simulink model "Aero2_Workspace"  (R2023a)
settings: Solver=ode4  StartTime=0.0  StopTime=inf  FixedStep=0.001  RelTol=1e-3  EnableMultiTasking=on
model workspace (MAT data in the model file):
  Dp = 0.001964
  Dt = 0.16743
  Dy = 0.001776
  Fc_p = 0
  Fc_y = 0.000919
  Jm = 4e-06
  Jp = 0.02318850045
  Jr = 4.4030375e-05
  Jr_p = 1.626e-05
  Jy = 0.02381041595
  Ka_p = 2.054e-06
  Ka_y = 1.1752e-06
  Ksp = 0.012956
  Rm = 10.6
  Sig = Simulink.Signal
  Sig.DataType = 'auto'
  Sig.Dimensions = -1
  Sig.DimensionsMode = 'auto'
  Sig.Complexity = 'auto'
  Sig.SampleTime = -1
  Sig.SamplingMode = 'auto'
  km = 0.04
  kt = 0.04
undefined symbols (not defined in the file or in its folder): qc_get_step_size
libraries: quarc_library x10, simulink x4
settings Model: SimulationMode=external  ExtModeTrigDuration=10000  Creator=mbohra  LastModifiedBy=Derek
settings SolverCC: AlgebraicLoopSolver=TrustRegion  PositivePriorityOrder=on
settings DataIOCC: ReturnWorkspaceOutputs=off
settings OptimizationCC: ReuseModelBlockBuffer=off
settings DebuggingCC: UnconnectedInputMsg=warning  UnconnectedOutputMsg=warning  UnconnectedLineMsg=warning  ArithmeticOperatorsInVariantConditions=warning
settings ModelReferenceCC: EnableRefExpFcnMdlSchedulingChecks=on
settings SFSimCC: SimUseLocalCustomCode=off  CustomCodeUndefinedFunction=UseInterfaceOnly
settings RTWCC: Description=QUARC Win64 Target Using Toolchain  SystemTargetFile=quarc_win64.tlc  TemplateMakefile=quarc_default_tmf  PostCodeGenCommand=packNGo(buildInfo, 'packType', 'hierarchical')  RTWUseLocalCustomCode=off  Toolchain=QUARC win64 | nmake (64-bit Windows)  BuildConfiguration=Faster Runs  DLArmComputeVersion=19.05
settings CodeAppCC: StateflowObjectComments=on
settings STFCustomTargetCC: SystemTargetFile=quarc_win64.tlc
settings GRTTargetCC: ParMdlRefBuildCompliant=off  CompOptLevelCompliant=off  CombineOutputUpdateFcns=off  MatFileLogging=off  CPPClassGenCompliant=off  GRTInterface=on  ExtMode=on  ExtModeMexFile=quarc_comm
settings ConfigComp: CovMetricSettings=dswe

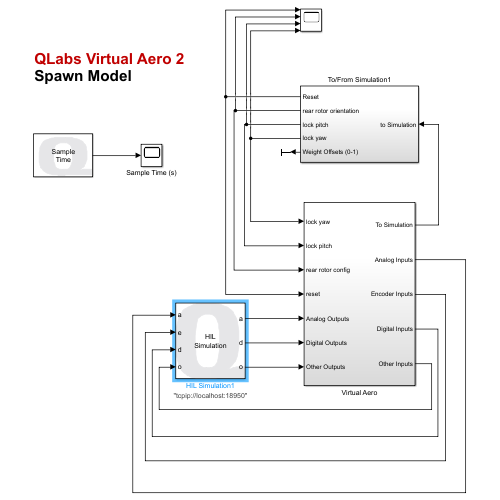
[thumbnail: Simulink's stored preview of the top-level diagram]
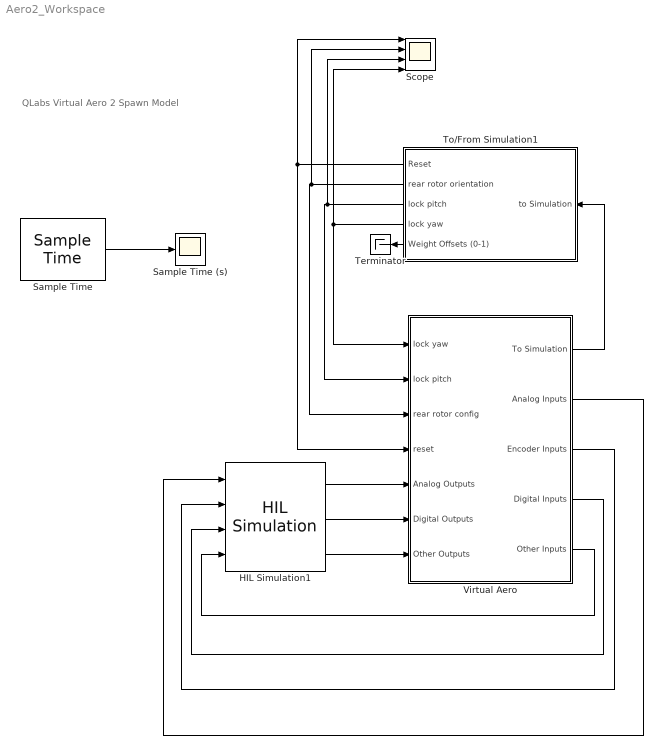
== system Aero2_Workspace ==
  note: QLabs Virtual Aero 2
      | Spawn Model
  HIL Simulation1 : quarc_library/Data Acquisition/Generic/Configuration/HIL Simulation  uri_source=Specify via dialog (do not evaluate)  uri=tcpip://localhost:18950  board_type=quanser_aero2_usb  board_id=0  sample_time=qc_get_step_size  active=on  num_clocks=1  num_interrupts=0  num_analog_inputs=2  num_analog_outputs=2  initial_analog=[]  num_digital_io=0  num_digital_inputs=3  num_digital_outputs=2  initial_digital=[1 1]  num_encoder_inputs=4  num_pwm_outputs=0  initial_pwm=[]  other_inputs=[3000:3002 4000:4002 14000:14003]  other_outputs=[11000:11002]  initial_other=[]  integer_get_property_codes=[]  double_get_property_codes=[]  string_get_property_codes=[]  integer_set_property_codes=[]  double_set_property_codes=[]  string_set_property_codes=[]  initial_integer_properties=0  initial_double_properties=0  initial_string_properties=[]  max_string_property=80  use_variable_size_strings=off
      settings: AttributesFormatString="\"tcpip://localhost:18950\""  SourceProductName=QUARC Targets
  Sample Time : quarc_library/Sources/Time/Sample Time  Priority=-99  sample_time=qc_get_step_size
  Sample Time (s) : Scope
  Scope : Scope  NumInputPorts=4
  Terminator : Terminator
  To/From Simulation1 : Subsystem
  Virtual Aero : Subsystem
  wires:
  HIL Simulation1/1 -> Virtual Aero/5(Analog Outputs)
  HIL Simulation1/2 -> Virtual Aero/6(Digital Outputs)
  HIL Simulation1/3 -> Virtual Aero/7(Other Outputs)
  Virtual Aero/5(Other Inputs) -> HIL Simulation1/4
  Virtual Aero/3(Encoder Inputs) -> HIL Simulation1/2
  Virtual Aero/2(Analog Inputs) -> HIL Simulation1/1
  To/From Simulation1/4(lock yaw) -> Virtual Aero/1(lock yaw), Scope/4
  To/From Simulation1/3(lock pitch) -> Scope/3, Virtual Aero/2(lock pitch)
  To/From Simulation1/1(Reset) -> Scope/1, Virtual Aero/4(reset)
  To/From Simulation1/2(rear rotor orientation) -> Scope/2, Virtual Aero/3(rear rotor config)
  Sample Time/1 -> Sample Time (s)/1
  Virtual Aero/1(To Simulation) -> To/From Simulation1/1(to Simulation)
  To/From Simulation1/5(Weight Offsets (0-1)) -> Terminator/1
  Virtual Aero/4(Digital Inputs) -> HIL Simulation1/3

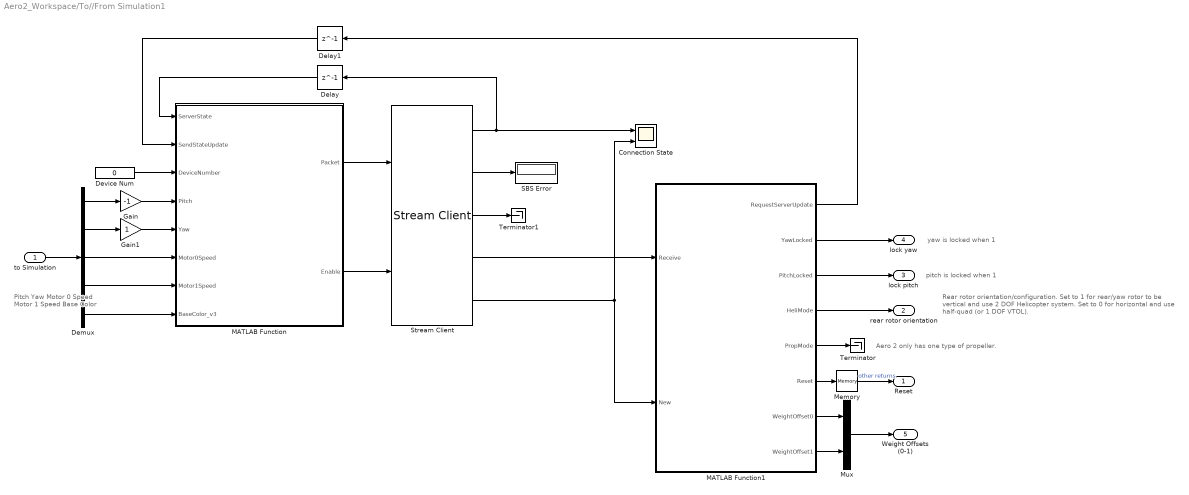
== system Aero2_Workspace/To//From Simulation1 ==
  note: Aero 2 only has one type of propeller.
  note: pitch is locked when 1
  note: Pitch
      | Yaw
      | Motor 0 Speed
      | Motor 1 Speed
      | Base Color
  note: Rear rotor orientation/configuration.
      | Set to 1 for rear/yaw rotor to be vertical and use 2 DOF Helicopter system.
      | Set to 0 for horizontal and use half-quad (or 1 DOF VTOL).
  note: yaw is locked when 1
  to Simulation : Inport
  "Connection State " : Scope  NumInputPorts=2
  Delay : Delay  DelayLength=1
  Delay1 : Delay  DelayLength=1
  Demux : Demux  Outputs=[1 1 1 1 3]
  Device Num : Constant  Value=0
  Gain : Gain  Gain=-1
  Gain1 : Gain
  MATLAB Function : MATLAB Function  TreatAsAtomicUnit=on
  MATLAB Function1 : MATLAB Function  TreatAsAtomicUnit=on
  Memory : Memory
  Mux : Mux  Inputs=2
  SBS Error : Display
      settings: Decimation=20
  Stream Client : quarc_library/Communications/Basic/Stream Client  uri_source=Specify via dialog (do not evaluate)  uri=tcpip://localhost:18000?nagle='off'  send_buffer_size=65537  receive_buffer_size=65537  byte_order=little endian (Intel - LSB first)  optimization=Minimum latency  send_options=Send all data  receive_options=Receive all data  default_value=[0]  sample_time=qc_get_step_size  active=off  implementation=Use blocking I/O in a separate thread  send_fifo_size=3  receive_fifo_size=3  send_priority=0  receive_priority=0  send_dimensions=on  receive_dimensions=on  max_dimensions=65537  data_type=uint8  type_expr=BusObject
      settings: AttributesFormatString="\"tcpip://localhost:18000?nagle='off'\""
  Terminator : Terminator
  Terminator1 : Terminator
  Reset : Outport  VectorParamsAs1DForOutWhenUnconnected=off
  rear rotor orientation : Outport  Port=2  VectorParamsAs1DForOutWhenUnconnected=off
  lock pitch : Outport  Port=3  VectorParamsAs1DForOutWhenUnconnected=off
  lock yaw : Outport  Port=4  VectorParamsAs1DForOutWhenUnconnected=off
  Weight Offsets (0-1) : Outport  Port=5  OutDataTypeStr=double  VectorParamsAs1DForOutWhenUnconnected=off
  wires:
  MATLAB Function1/3(PitchLocked) -> lock pitch/1
  MATLAB Function1/2(YawLocked) -> lock yaw/1
  MATLAB Function1/4(HeliMode) -> rear rotor orientation/1
  MATLAB Function/1(Packet) -> Stream Client/1
  Stream Client/5 -> MATLAB Function1/2(New), "Connection State "/2
  Stream Client/2 -> SBS Error/1
  Demux/5 -> MATLAB Function/8(BaseColor_v3)
  Stream Client/4 -> MATLAB Function1/1(Receive)
  Stream Client/3 -> Terminator1/1
  Demux/4 -> MATLAB Function/7(Motor1Speed)
  MATLAB Function/2(Enable) -> Stream Client/2
  Demux/3 -> MATLAB Function/6(Motor0Speed)
  MATLAB Function1/1(RequestServerUpdate) -> Delay1/1
  to Simulation/1 -> Demux/1
  Delay1/1 -> MATLAB Function/2(SendStateUpdate)
  Stream Client/1 -> Delay/1, "Connection State "/1
  Delay/1 -> MATLAB Function/1(ServerState)
  Device Num/1 -> MATLAB Function/3(DeviceNumber)
  Demux/1 -> Gain/1
  Demux/2 -> Gain1/1
  MATLAB Function1/6(Reset) -> Memory/1
  MATLAB Function1/5(PropMode) -> Terminator/1
  Mux/1 -> Weight Offsets (0-1)/1
  MATLAB Function1/7(WeightOffset0) -> Mux/1
  MATLAB Function1/8(WeightOffset1) -> Mux/2
  Memory/1 -> Reset/1  "other returns"
  Gain/1 -> MATLAB Function/4(Pitch)
  Gain1/1 -> MATLAB Function/5(Yaw)

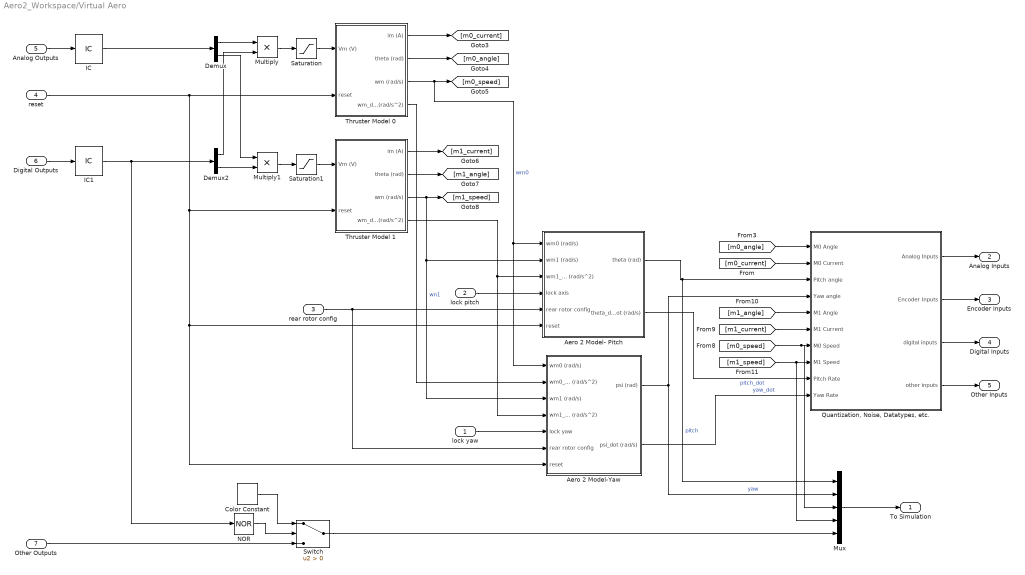
== system Aero2_Workspace/Virtual Aero ==
  lock yaw : Inport
  lock pitch : Inport  Port=2
  rear rotor config : Inport  Port=3
  reset : Inport  Port=4
  Analog Outputs : Inport  Port=5
  Digital Outputs : Inport  Port=6
  Other Outputs : Inport  Port=7
  Aero 2 Model- Pitch : Subsystem
  Aero 2 Model-Yaw : Subsystem
  Color Constant : quarc_library/Sources/Signals/Color Constant  color=[1 0 0]
      settings: SourceProductName=QUARC Targets
  Demux : Demux  Outputs=2
  Demux2 : Demux  Outputs=2
  IC : InitialCondition  Value=0
  IC1 : InitialCondition  Value=0
  Multiply : Product
  Multiply1 : Product
  Mux : Mux  Inputs=5
  NOR : Logic  Operator=NOR  Inputs=1  IconShape=distinctive  AllPortsSameDT=off  OutDataTypeStr=boolean
  "Quantization, Noise, Datatypes, etc." : Subsystem
  Saturation : Saturate  UpperLimit=24  LowerLimit=-24
  Saturation1 : Saturate  UpperLimit=24  LowerLimit=-24
  Switch : Switch  Criteria=u2 > Threshold  SaturateOnIntegerOverflow=off  InputSameDT=off
  Thruster Model 0 : Subsystem
  Thruster Model 1 : Subsystem
  To Simulation : Outport  VectorParamsAs1DForOutWhenUnconnected=off
  Analog Inputs : Outport  Port=2  VectorParamsAs1DForOutWhenUnconnected=off
  Encoder Inputs : Outport  Port=3  VectorParamsAs1DForOutWhenUnconnected=off
  Digital Inputs : Outport  Port=4  VectorParamsAs1DForOutWhenUnconnected=off
  Other Inputs : Outport  Port=5  VectorParamsAs1DForOutWhenUnconnected=off
  wires:
  Analog Outputs/1 -> IC/1
  Digital Outputs/1 -> IC1/1
  Demux/1 -> Multiply/1
  Demux2/1 -> Multiply/2
  Demux/2 -> Multiply1/1
  Demux2/2 -> Multiply1/2
  "Quantization, Noise, Datatypes, etc."/1(Analog Inputs) -> Analog Inputs/1
  "Quantization, Noise, Datatypes, etc."/2(Encoder Inputs) -> Encoder Inputs/1
  "Quantization, Noise, Datatypes, etc."/4(other inputs) -> Other Inputs/1
  Thruster Model 0/1(im (A)) -> [m0_current]
  Thruster Model 0/2(theta (rad)) -> [m0_angle]
  Thruster Model 0/3(wm (rad/s)) -> [m0_speed], Aero 2 Model-Yaw/1(wm0 (rad/s)), Aero 2 Model- Pitch/1(wm0 (rad/s))  "wm0"
  [m0_current] -> "Quantization, Noise, Datatypes, etc."/2(M0 Current)
  [m0_angle] -> "Quantization, Noise, Datatypes, etc."/1(M0 Angle)
  [m0_speed] -> Mux/3, "Quantization, Noise, Datatypes, etc."/7(M0 Speed)
  [m1_speed] -> "Quantization, Noise, Datatypes, etc."/8(M1 Speed), Mux/4
  [m1_angle] -> "Quantization, Noise, Datatypes, etc."/5(M1 Angle)
  [m1_current] -> "Quantization, Noise, Datatypes, etc."/6(M1 Current)
  Aero 2 Model-Yaw/1(psi (rad)) -> "Quantization, Noise, Datatypes, etc."/4(Yaw angle), Mux/2  "yaw"
  Thruster Model 1/1(im (A)) -> [m1_current]
  Thruster Model 1/2(theta (rad)) -> [m1_angle]
  Thruster Model 1/3(wm (rad/s)) -> Aero 2 Model-Yaw/3(wm1 (rad/s)), Aero 2 Model- Pitch/2(wm1 (rad/s)), [m1_speed]  "wn1"
  Thruster Model 0/4(wm_dot (rad/s^2)) -> Aero 2 Model-Yaw/2(wm0_dot (rad/s^2))
  Aero 2 Model-Yaw/2(psi_dot (rad/s)) -> "Quantization, Noise, Datatypes, etc."/10(Yaw Rate)  "yaw_dot"
  Thruster Model 1/4(wm_dot (rad/s^2)) -> Aero 2 Model-Yaw/4(wm1_dot (rad/s^2)), Aero 2 Model- Pitch/3(wm1_dot (rad/s^2))
  lock yaw/1 -> Aero 2 Model-Yaw/5(lock yaw)
  lock pitch/1 -> Aero 2 Model- Pitch/4(lock axis)
  reset/1 -> Thruster Model 1/2(reset), Aero 2 Model- Pitch/6(reset), Aero 2 Model-Yaw/7(reset), Thruster Model 0/2(reset)
  rear rotor config/1 -> Aero 2 Model-Yaw/6(rear rotor config), Aero 2 Model- Pitch/5(rear rotor config)
  IC1/1 -> Demux2/1, NOR/1
  Multiply/1 -> Saturation/1
  Saturation/1 -> Thruster Model 0/1(Vm (V))
  Multiply1/1 -> Saturation1/1
  Saturation1/1 -> Thruster Model 1/1(Vm (V))
  Aero 2 Model- Pitch/1(theta (rad)) -> Mux/1, "Quantization, Noise, Datatypes, etc."/3(Pitch angle)  "pitch"
  Aero 2 Model- Pitch/2(theta_dot (rad/s)) -> "Quantization, Noise, Datatypes, etc."/9(Pitch Rate)  "pitch_dot"
  Mux/1 -> To Simulation/1
  "Quantization, Noise, Datatypes, etc."/3(digital inputs) -> Digital Inputs/1
  Color Constant/1 -> Switch/1
  NOR/1 -> Switch/2
  Other Outputs/1 -> Switch/3
  Switch/1 -> Mux/5
  IC/1 -> Demux/1

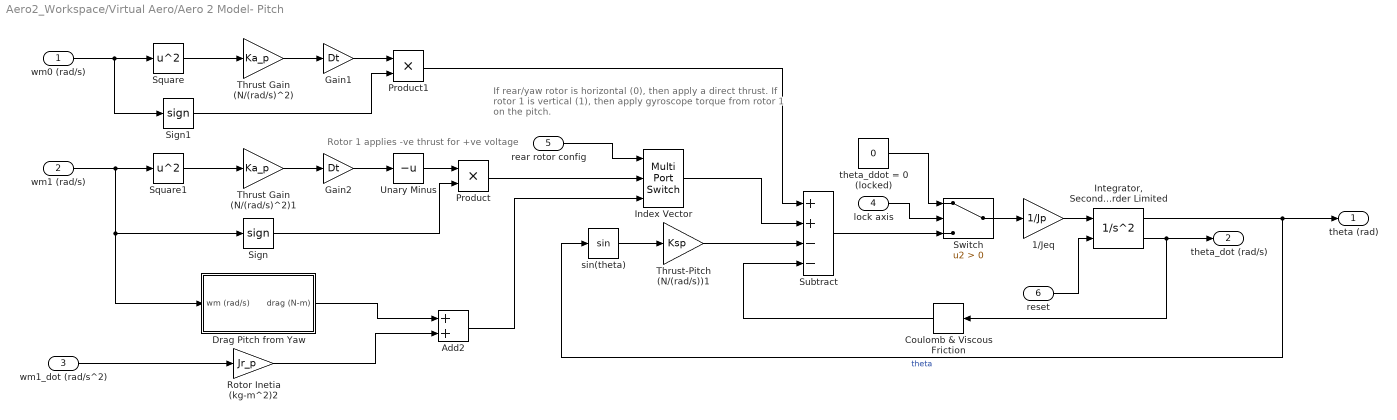
== system Aero2_Workspace/Virtual Aero/Aero 2 Model- Pitch ==
  note: If rear/yaw rotor is horizontal (0), then apply a direct thrust.
      | If rotor 1 is vertical (1), then apply gyroscope torque from rotor 1 on the pitch.
  note: Rotor 1 applies -ve thrust for +ve voltage
  wm0 (rad/s) : Inport
  wm1 (rad/s) : Inport  Port=2
  wm1_dot (rad/s^2) : Inport  Port=3
  lock axis : Inport  Port=4
  rear rotor config : Inport  Port=5
  reset : Inport  Port=6
  1/Jeq : Gain  Gain=1/Jp
  Add2 : Sum
  Coulomb & Viscous Friction : simulink/Discontinuities/Coulomb & Viscous Friction  offset=Fc_p  gain=Dp
  Drag Pitch from Yaw : Subsystem
  Gain1 : Gain  Gain=Dt
  Gain2 : Gain  Gain=Dt
  Index Vector : MultiPortSwitch  DataPortOrder=Zero-based contiguous  Inputs=2  zeroidx=on  SaturateOnIntegerOverflow=off  InputSameDT=off
  "Integrator, Second-Order Limited" : SecondOrderIntegrator  LimitX=on  UpperLimitX=0.85  LowerLimitX=-0.85  ExternalReset=rising  ReinitDXDTwhenXreachesSaturation=on
  Product : Product
  Product1 : Product
  Rotor Inetia (kg-m^2)2 : Gain  Gain=Jr_p
  Sign : Signum
  Sign1 : Signum
  Square : Math  Operator=square
  Square1 : Math  Operator=square
  Subtract : Sum  Inputs=++--
  Switch : Switch  Criteria=u2 > Threshold  SaturateOnIntegerOverflow=off  InputSameDT=off
  Thrust Gain (N/(rad/s)^2) : Gain  Gain=Ka_p
  Thrust Gain (N/(rad/s)^2)1 : Gain  Gain=Ka_p
  Thrust-Pitch (N/(rad/s))1 : Gain  Gain=Ksp
  Unary Minus : UnaryMinus
  sin(theta) : Trigonometry
  theta_ddot = 0 (locked) : Constant  Value=0
  theta (rad) : Outport
  theta_dot (rad/s) : Outport  Port=2
  wires:
  Drag Pitch from Yaw/1(drag (N-m)) -> Add2/1
  Add2/1 -> Index Vector/3
  "Integrator, Second-Order Limited"/2 -> theta_dot (rad/s)/1, Coulomb & Viscous Friction/1
  Unary Minus/1 -> Product/1
  Product/1 -> Index Vector/2
  rear rotor config/1 -> Index Vector/1
  Sign/1 -> Product/2
  Gain2/1 -> Unary Minus/1
  Thrust Gain (N/(rad/s)^2)1/1 -> Gain2/1
  Square1/1 -> Thrust Gain (N/(rad/s)^2)1/1
  wm1 (rad/s)/1 -> Square1/1, Sign/1, Drag Pitch from Yaw/1(wm (rad/s))
  Thrust-Pitch (N/(rad/s))1/1 -> Subtract/3
  Coulomb & Viscous Friction/1 -> Subtract/4
  wm1_dot (rad/s^2)/1 -> Rotor Inetia (kg-m^2)2/1
  Rotor Inetia (kg-m^2)2/1 -> Add2/2
  theta_ddot = 0 (locked)/1 -> Switch/1
  Switch/1 -> 1/Jeq/1
  Subtract/1 -> Switch/3
  lock axis/1 -> Switch/2
  sin(theta)/1 -> Thrust-Pitch (N/(rad/s))1/1
  Thrust Gain (N/(rad/s)^2)/1 -> Gain1/1
  Square/1 -> Thrust Gain (N/(rad/s)^2)/1
  wm0 (rad/s)/1 -> Sign1/1, Square/1
  1/Jeq/1 -> "Integrator, Second-Order Limited"/1
  "Integrator, Second-Order Limited"/1 -> theta (rad)/1, sin(theta)/1  "theta"
  reset/1 -> "Integrator, Second-Order Limited"/2
  Sign1/1 -> Product1/2
  Gain1/1 -> Product1/1
  Product1/1 -> Subtract/1
  Index Vector/1 -> Subtract/2

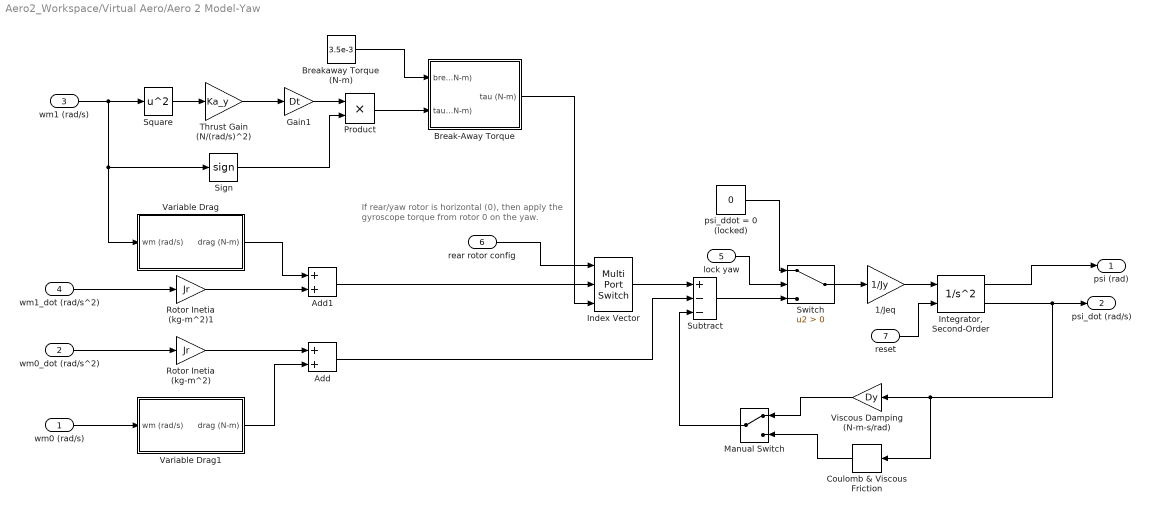
== system Aero2_Workspace/Virtual Aero/Aero 2 Model-Yaw ==
  note: If rear/yaw rotor is horizontal (0), then apply the gyroscope torque from rotor 0 on the yaw.
  wm0 (rad/s) : Inport
  wm0_dot (rad/s^2) : Inport  Port=2
  wm1 (rad/s) : Inport  Port=3
  wm1_dot (rad/s^2) : Inport  Port=4
  lock yaw : Inport  Port=5
  rear rotor config : Inport  Port=6
  reset : Inport  Port=7
  1/Jeq : Gain  Gain=1/Jy
  Add : Sum
  Add1 : Sum
  Break-Away Torque : Subsystem
  Breakaway Torque (N-m) : Constant  Value=3.5e-3
  Coulomb & Viscous Friction : simulink/Discontinuities/Coulomb & Viscous Friction  offset=Fc_y  gain=Dy
  Gain1 : Gain  Gain=Dt
  Index Vector : MultiPortSwitch  DataPortOrder=Zero-based contiguous  Inputs=2  zeroidx=on  SaturateOnIntegerOverflow=off  InputSameDT=off
  "Integrator, Second-Order" : SecondOrderIntegrator  ExternalReset=rising
  Manual Switch : ManualSwitch
  Product : Product
  Rotor Inetia (kg-m^2) : Gain  Gain=Jr
  Rotor Inetia (kg-m^2)1 : Gain  Gain=Jr
  Sign : Signum
  Square : Math  Operator=square
  Subtract : Sum  Inputs=+--
  Switch : Switch  Criteria=u2 > Threshold  SaturateOnIntegerOverflow=off  InputSameDT=off
  Thrust Gain (N/(rad/s)^2) : Gain  Gain=Ka_y
  Variable Drag : Subsystem
  Variable Drag1 : Subsystem
  Viscous Damping (N-m-s/rad) : Gain  Gain=Dy
  psi_ddot = 0 (locked) : Constant  Value=0
  psi (rad) : Outport
  psi_dot (rad/s) : Outport  Port=2
  wires:
  Add/1 -> Subtract/2
  Add1/1 -> Index Vector/2
  Break-Away Torque/1(tau (N-m)) -> Index Vector/3
  lock yaw/1 -> Switch/2
  Switch/1 -> 1/Jeq/1
  Subtract/1 -> Switch/3
  psi_ddot = 0 (locked)/1 -> Switch/1
  Thrust Gain (N/(rad/s)^2)/1 -> Gain1/1
  Square/1 -> Thrust Gain (N/(rad/s)^2)/1
  wm1 (rad/s)/1 -> Square/1, Sign/1, Variable Drag/1(wm (rad/s))
  1/Jeq/1 -> "Integrator, Second-Order"/1
  wm0_dot (rad/s^2)/1 -> Rotor Inetia (kg-m^2)/1
  wm1_dot (rad/s^2)/1 -> Rotor Inetia (kg-m^2)1/1
  Rotor Inetia (kg-m^2)1/1 -> Add1/2
  rear rotor config/1 -> Index Vector/1
  Breakaway Torque (N-m)/1 -> Break-Away Torque/1(breakaway (N-m))
  Rotor Inetia (kg-m^2)/1 -> Add/1
  Index Vector/1 -> Subtract/1
  Variable Drag/1(drag (N-m)) -> Add1/1
  wm0 (rad/s)/1 -> Variable Drag1/1(wm (rad/s))
  Variable Drag1/1(drag (N-m)) -> Add/2
  "Integrator, Second-Order"/2 -> psi_dot (rad/s)/1, Viscous Damping (N-m-s/rad)/1, Coulomb & Viscous Friction/1
  "Integrator, Second-Order"/1 -> psi (rad)/1
  Manual Switch/1 -> Subtract/3
  reset/1 -> "Integrator, Second-Order"/2
  Gain1/1 -> Product/1
  Product/1 -> Break-Away Torque/2(tau_a (N-m))
  Sign/1 -> Product/2
  Viscous Damping (N-m-s/rad)/1 -> Manual Switch/1
  Coulomb & Viscous Friction/1 -> Manual Switch/2

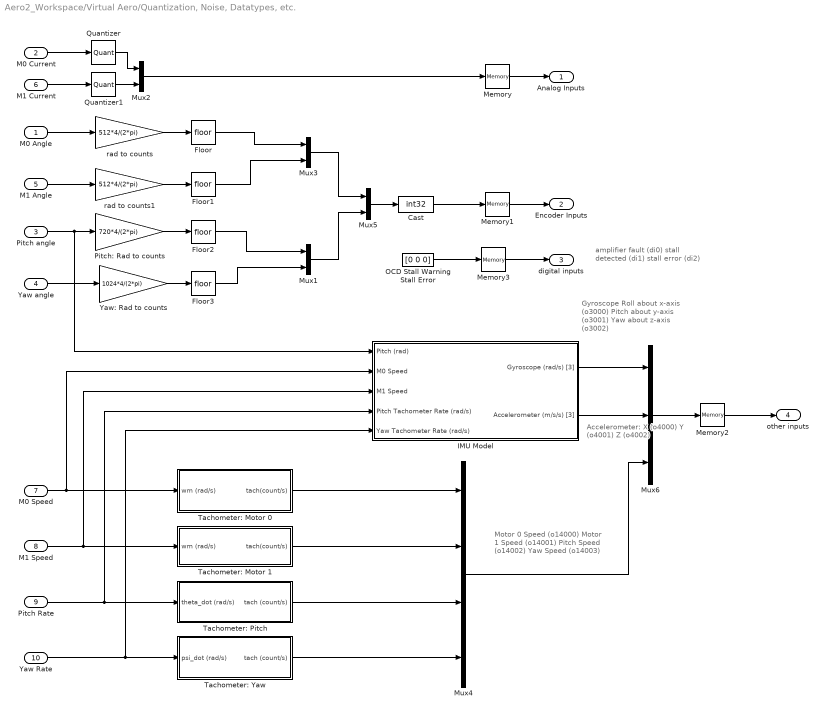
== system Aero2_Workspace/Virtual Aero/Quantization, Noise, Datatypes, etc. ==
  note: Motor 0 Speed (o14000)
      | Motor 1 Speed (o14001)
      | Pitch Speed (o14002)
      | Yaw Speed (o14003)
  note: Gyroscope
      | Roll about x-axis (o3000)
      | Pitch about y-axis (o3001)
      | Yaw about z-axis (o3002)
  note: Accelerometer:
      | X (o4000)
      | Y (o4001)
      | Z (o4002)
  note: amplifier fault (di0)
      | stall detected (di1)
      | stall error (di2)
  M0 Angle : Inport
  M0 Current : Inport  Port=2
  Pitch angle : Inport  Port=3
  Yaw angle : Inport  Port=4
  M1 Angle : Inport  Port=5
  M1 Current : Inport  Port=6
  M0 Speed : Inport  Port=7
  M1 Speed : Inport  Port=8
  Pitch Rate : Inport  Port=9
  Yaw Rate : Inport  Port=10
  Cast : DataTypeConversion  OutDataTypeStr=int32  SaturateOnIntegerOverflow=off  RndMeth=Floor
  Floor{,1..3} (4 alike) : Rounding
  IMU Model : Subsystem
  Memory{,1..3} (4 alike) : quarc_library/Discrete/Memory  initial_condition=0  sample_time=-1
      settings: SourceProductName=QUARC Targets
  Mux{1..3,5} (4 alike) : Mux  Inputs=2
  Mux4 : Mux
  Mux6 : Mux  Inputs=3
  OCD Stall Warning Stall Error : Constant  Value=[0 0 0]  OutDataTypeStr=boolean
  Pitch: Rad to counts : Gain  Gain=720*4/(2*pi)
  Quantizer : Quantizer  QuantizationInterval=1/9828
  Quantizer1 : Quantizer  QuantizationInterval=1/9828
  Tachometer: Motor 0 : Subsystem
  Tachometer: Motor 1 : Subsystem
  Tachometer: Pitch : Subsystem
  Tachometer: Yaw : Subsystem
  Yaw: Rad to counts : Gain  Gain=1024*4/(2*pi)
  rad to counts : Gain  Gain=512*4/(2*pi)
  rad to counts1 : Gain  Gain=512*4/(2*pi)
  Analog Inputs : Outport  VectorParamsAs1DForOutWhenUnconnected=off
  Encoder Inputs : Outport  Port=2  VectorParamsAs1DForOutWhenUnconnected=off
  digital inputs : Outport  Port=3
  other inputs : Outport  Port=4  VectorParamsAs1DForOutWhenUnconnected=off
  wires:
  Cast/1 -> Memory1/1
  Yaw: Rad to counts/1 -> Floor3/1
  Yaw angle/1 -> Yaw: Rad to counts/1
  Pitch angle/1 -> IMU Model/1("Pitch (rad) "), Pitch: Rad to counts/1
  Pitch: Rad to counts/1 -> Floor2/1
  Mux1/1 -> Mux5/2
  Floor/1 -> Mux3/1
  Memory/1 -> Analog Inputs/1
  M1 Angle/1 -> rad to counts1/1
  Mux3/1 -> Mux5/1
  Mux5/1 -> Cast/1
  Mux2/1 -> Memory/1
  M0 Current/1 -> Quantizer/1
  Memory1/1 -> Encoder Inputs/1
  M1 Current/1 -> Quantizer1/1
  M0 Angle/1 -> rad to counts/1
  rad to counts/1 -> Floor/1
  Floor1/1 -> Mux3/2
  rad to counts1/1 -> Floor1/1
  Tachometer: Motor 1/1(tach(count/s)) -> Mux4/2
  M1 Speed/1 -> IMU Model/3(M1 Speed), Tachometer: Motor 1/1(wm (rad/s))
  Quantizer/1 -> Mux2/1
  Quantizer1/1 -> Mux2/2
  M0 Speed/1 -> IMU Model/2(M0 Speed), Tachometer: Motor 0/1(wm (rad/s))
  Tachometer: Motor 0/1(tach(count/s)) -> Mux4/1
  Pitch Rate/1 -> IMU Model/4(Pitch Tachometer Rate (rad/s)), Tachometer: Pitch/1(theta_dot (rad/s))
  Tachometer: Pitch/1(tach (count/s)) -> Mux4/3
  Yaw Rate/1 -> IMU Model/5(Yaw Tachometer Rate (rad/s)), Tachometer: Yaw/1(psi_dot (rad/s))
  Tachometer: Yaw/1(tach (count/s)) -> Mux4/4
  IMU Model/1(Gyroscope (rad/s) [3]) -> Mux6/1
  IMU Model/2(Accelerometer (m/s/s) [3]) -> Mux6/2
  Mux4/1 -> Mux6/3
  Mux6/1 -> Memory2/1
  Memory2/1 -> other inputs/1
  Floor2/1 -> Mux1/1
  Floor3/1 -> Mux1/2
  OCD Stall Warning Stall Error/1 -> Memory3/1
  Memory3/1 -> digital inputs/1

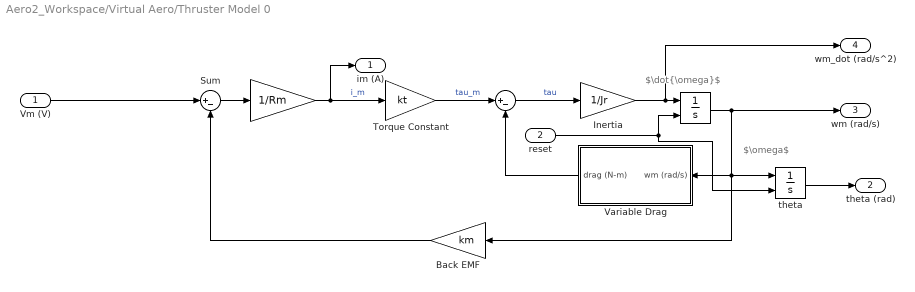
== system Aero2_Workspace/Virtual Aero/Thruster Model 0 ==
  note: $\dot{\omega}$
  note: $\omega$
  Vm (V) : Inport
  reset : Inport  Port=2
  " " : Integrator  ExternalReset=rising
  "  " : Gain  Gain=1/Rm  SaturateOnIntegerOverflow=on  OutDataTypeStr=Inherit: Same as input  ParamDataTypeStr=Inherit: Same as input
  "   " : Sum  Inputs=|+-
  " theta" : Integrator  ExternalReset=rising
  Back EMF : Gain  Gain=km
  Inertia : Gain  Gain=1/Jr
  Sum : Sum  Inputs=|+-  InputSameDT=on  SaturateOnIntegerOverflow=on  OutDataTypeStr=Inherit: Same as first input
  Torque Constant : Gain  Gain=kt
  Variable Drag : Subsystem
  im (A) : Outport
  theta (rad) : Outport  Port=2
  wm (rad/s) : Outport  Port=3
  wm_dot (rad/s^2) : Outport  Port=4
  wires:
  " theta"/1 -> theta (rad)/1
  Inertia/1 -> wm_dot (rad/s^2)/1, " "/1
  "   "/1 -> Inertia/1  "tau"
  Torque Constant/1 -> "   "/1  "tau_m"
  Back EMF/1 -> Sum/2
  Sum/1 -> "  "/1
  Vm (V)/1 -> Sum/1
  "  "/1 -> im (A)/1, Torque Constant/1  "i_m"
  " "/1 -> wm (rad/s)/1, Variable Drag/1(wm (rad/s)), Back EMF/1, " theta"/1
  Variable Drag/1(drag (N-m)) -> "   "/2
  reset/1 -> " theta"/2, " "/2

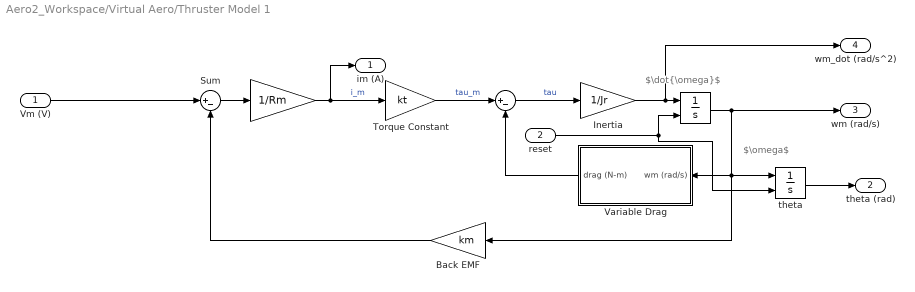
== system Aero2_Workspace/Virtual Aero/Thruster Model 1 ==
  note: $\omega$
  note: $\dot{\omega}$
  Vm (V) : Inport
  reset : Inport  Port=2
  " " : Integrator  ExternalReset=rising
  "  " : Gain  Gain=1/Rm  SaturateOnIntegerOverflow=on  OutDataTypeStr=Inherit: Same as input  ParamDataTypeStr=Inherit: Same as input
  "   " : Sum  Inputs=|+-
  " theta" : Integrator  ExternalReset=rising
  Back EMF : Gain  Gain=km
  Inertia : Gain  Gain=1/Jr
  Sum : Sum  Inputs=|+-  InputSameDT=on  SaturateOnIntegerOverflow=on  OutDataTypeStr=Inherit: Same as first input
  Torque Constant : Gain  Gain=kt
  Variable Drag : Subsystem
  im (A) : Outport
  theta (rad) : Outport  Port=2
  wm (rad/s) : Outport  Port=3
  wm_dot (rad/s^2) : Outport  Port=4
  wires:
  reset/1 -> " "/2, " theta"/2
  Variable Drag/1(drag (N-m)) -> "   "/2
  " "/1 -> Variable Drag/1(wm (rad/s)), " theta"/1, Back EMF/1, wm (rad/s)/1
  "  "/1 -> Torque Constant/1, im (A)/1  "i_m"
  Vm (V)/1 -> Sum/1
  Sum/1 -> "  "/1
  Back EMF/1 -> Sum/2
  Torque Constant/1 -> "   "/1  "tau_m"
  "   "/1 -> Inertia/1  "tau"
  Inertia/1 -> " "/1, wm_dot (rad/s^2)/1
  " theta"/1 -> theta (rad)/1

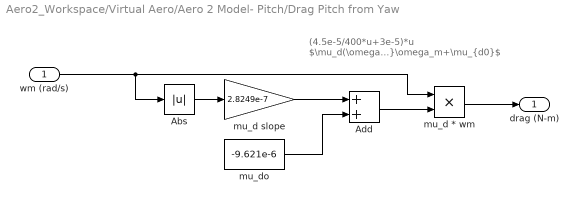
== system Aero2_Workspace/Virtual Aero/Aero 2 Model- Pitch/Drag Pitch from Yaw ==
  note: (4.5e-5/400*u+3e-5)*u
      | $\mu_d(\omega_m)=\mu_{d,slope}\omega_m+\mu_{d0}$
  wm (rad/s) : Inport
  Abs : Abs  SaturateOnIntegerOverflow=off
  Add : Sum
  mu_d * wm : Product
  mu_d slope : Gain  Gain=2.8249e-7
  mu_do : Constant  Value=-9.621e-6
  drag (N-m) : Outport
  wires:
  wm (rad/s)/1 -> mu_d * wm/1, Abs/1
  Add/1 -> mu_d * wm/2
  mu_d slope/1 -> Add/1
  mu_d * wm/1 -> drag (N-m)/1
  mu_do/1 -> Add/2
  Abs/1 -> mu_d slope/1

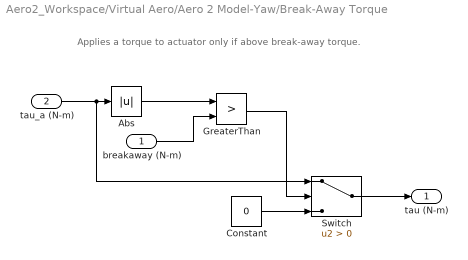
== system Aero2_Workspace/Virtual Aero/Aero 2 Model-Yaw/Break-Away Torque ==
  note: Applies a torque to actuator only if above break-away torque.
  breakaway (N-m) : Inport
  tau_a (N-m) : Inport  Port=2
  Abs : Abs  SaturateOnIntegerOverflow=off
  Constant : Constant  Value=0
  GreaterThan : RelationalOperator  Operator=>  OutDataTypeStr=boolean  RndMeth=Simplest  InputSameDT=off
  Switch : Switch  Criteria=u2 > Threshold  SaturateOnIntegerOverflow=off  InputSameDT=off
  tau (N-m) : Outport
  wires:
  Switch/1 -> tau (N-m)/1
  GreaterThan/1 -> Switch/2
  breakaway (N-m)/1 -> GreaterThan/2
  Constant/1 -> Switch/3
  tau_a (N-m)/1 -> Switch/1, Abs/1
  Abs/1 -> GreaterThan/1

== system Aero2_Workspace/Virtual Aero/Aero 2 Model-Yaw/Variable Drag ==
  note: (4.5e-5/400*u+3e-5)*u
      | $\mu_d(\omega_m)=\mu_{d,slope}\omega_m+\mu_{d0}$
  wm (rad/s) : Inport
  Abs : Abs  SaturateOnIntegerOverflow=off
  Add : Sum
  mu_d * wm : Product
  mu_d slope : Gain  Gain=8.649e-8
  mu_do : Constant  Value=-7.99e-6
  drag (N-m) : Outport
  wires:
  wm (rad/s)/1 -> mu_d * wm/1, Abs/1
  Add/1 -> mu_d * wm/2
  mu_d slope/1 -> Add/1
  mu_d * wm/1 -> drag (N-m)/1
  mu_do/1 -> Add/2
  Abs/1 -> mu_d slope/1

== system Aero2_Workspace/Virtual Aero/Aero 2 Model-Yaw/Variable Drag1 ==
  note: (4.5e-5/400*u+3e-5)*u
      | $\mu_d(\omega_m)=\mu_{d,slope}\omega_m+\mu_{d0}$
  wm (rad/s) : Inport
  Abs : Abs  SaturateOnIntegerOverflow=off
  Add : Sum
  mu_d * wm : Product
  mu_d slope : Gain  Gain=8.649e-8
  mu_do : Constant  Value=-7.99e-6
  drag (N-m) : Outport
  wires:
  Abs/1 -> mu_d slope/1
  mu_do/1 -> Add/2
  mu_d * wm/1 -> drag (N-m)/1
  mu_d slope/1 -> Add/1
  Add/1 -> mu_d * wm/2
  wm (rad/s)/1 -> Abs/1, mu_d * wm/1

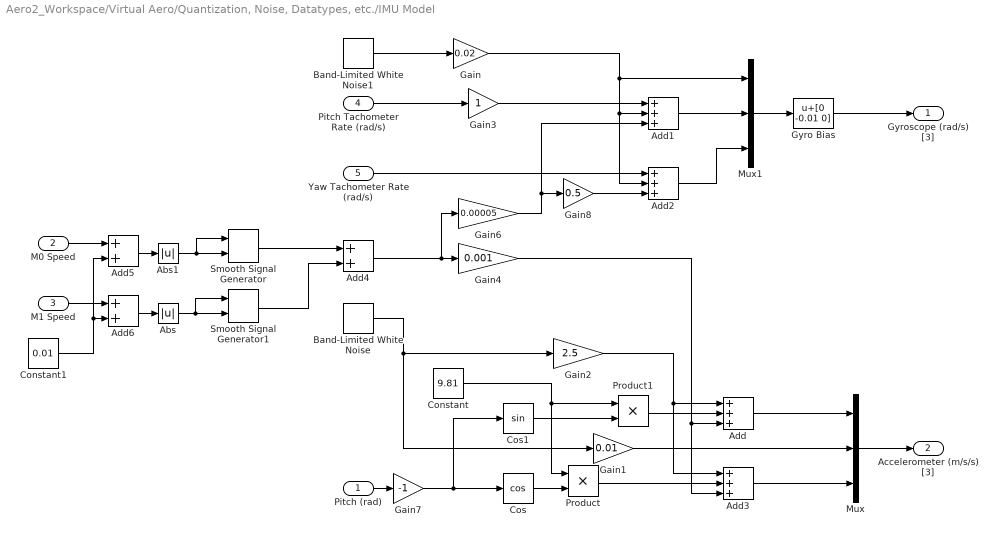
== system Aero2_Workspace/Virtual Aero/Quantization, Noise, Datatypes, etc./IMU Model ==
  "Pitch (rad) " : Inport
  M0 Speed : Inport  Port=2
  M1 Speed : Inport  Port=3
  Pitch Tachometer Rate (rad/s) : Inport  Port=4
  Yaw Tachometer Rate (rad/s) : Inport  Port=5
  Abs : Abs  SaturateOnIntegerOverflow=off
  Abs1 : Abs  SaturateOnIntegerOverflow=off
  Add{,1..3} (4 alike) : Sum  Inputs=+++
  Add4 : Sum
  Add5 : Sum
  Add6 : Sum
  Band-Limited White Noise : simulink/Sources/Band-Limited White Noise  Cov=[0.00001]  Ts=qc_get_step_size  seed=randi(10000, 1)
  Band-Limited White Noise1 : simulink/Sources/Band-Limited White Noise  Cov=[0.00001]  Ts=qc_get_step_size  seed=randi(10000, 1)
  Constant : Constant  Value=9.81
  Constant1 : Constant  Value=0.01
  Cos : Trigonometry  Operator=cos
  Cos1 : Trigonometry
  Gain : Gain  Gain=0.02
  Gain1 : Gain  Gain=0.01
  Gain2 : Gain  Gain=2.5
  Gain3 : Gain
  Gain4 : Gain  Gain=0.001
  Gain6 : Gain  Gain=0.00005
  Gain7 : Gain  Gain=-1
  Gain8 : Gain  Gain=0.5
  Gyro Bias : Bias  Bias=[0 -0.01 0]  SaturateOnIntegerOverflow=off
  Mux : Mux  Inputs=3
  Mux1 : Mux  Inputs=3
  Product : Product
  Product1 : Product
  Smooth Signal Generator : quarc_library/Sources/Signals/Smooth Signal Generator  signal_type=Sine  source=External (input ports)  amplitude=1  frequency=1  initial_phase=0  sample_time=qc_get_step_size  output_cos=off
      settings: SourceProductName=QUARC Targets
  Smooth Signal Generator1 : quarc_library/Sources/Signals/Smooth Signal Generator  signal_type=Sine  source=External (input ports)  amplitude=1  frequency=1  initial_phase=0  sample_time=qc_get_step_size  output_cos=off
      settings: SourceProductName=QUARC Targets
  Gyroscope (rad/s) [3] : Outport  VectorParamsAs1DForOutWhenUnconnected=off
  Accelerometer (m/s/s) [3] : Outport  Port=2  VectorParamsAs1DForOutWhenUnconnected=off
  wires:
  Gyro Bias/1 -> Gyroscope (rad/s) [3]/1
  Add1/1 -> Mux1/2
  Abs1/1 -> Smooth Signal Generator/2, Smooth Signal Generator/1
  Abs/1 -> Smooth Signal Generator1/2, Smooth Signal Generator1/1
  Add6/1 -> Abs/1
  Add5/1 -> Abs1/1
  Gain4/1 -> Add3/3, Add/3
  Gain6/1 -> Gain8/1, Add1/3
  Gain8/1 -> Add2/3
  M1 Speed/1 -> Add6/1
  Constant1/1 -> Add5/2, Add6/2
  M0 Speed/1 -> Add5/1
  Add4/1 -> Gain4/1, Gain6/1
  Smooth Signal Generator/1 -> Add4/1
  Smooth Signal Generator1/1 -> Add4/2
  Gain3/1 -> Add1/1
  Add3/1 -> Mux/3
  Product/1 -> Add3/2
  Product1/1 -> Add/2
  Gain1/1 -> Mux/2
  Mux1/1 -> Gyro Bias/1
  Pitch Tachometer Rate (rad/s)/1 -> Gain3/1
  Band-Limited White Noise1/1 -> Gain/1
  Band-Limited White Noise/1 -> Gain1/1, Gain2/1
  "Pitch (rad) "/1 -> Gain7/1
  Constant/1 -> Product1/1, Product/1
  Cos1/1 -> Product1/2
  Cos/1 -> Product/2
  Yaw Tachometer Rate (rad/s)/1 -> Add2/1
  Add2/1 -> Mux1/3
  Gain/1 -> Mux1/1, Add1/2, Add2/2
  Gain2/1 -> Add3/1, Add/1
  Mux/1 -> Accelerometer (m/s/s) [3]/1
  Add/1 -> Mux/1
  Gain7/1 -> Cos1/1, Cos/1

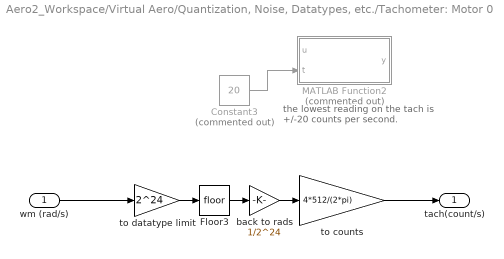
== system Aero2_Workspace/Virtual Aero/Quantization, Noise, Datatypes, etc./Tachometer: Motor 0 ==
  note: the lowest reading on the tach
      | is +/-20 counts per second.
  wm (rad/s) : Inport
  Constant3 : Constant  Commented=on  Value=20
  Floor3 : Rounding
  MATLAB Function2 : MATLAB Function  Commented=on  TreatAsAtomicUnit=on
  back to rads : Gain  Gain=1/2^24
  to counts : Gain  Gain=4*512/(2*pi)
  to datatype limit : Gain  Gain=2^24
  tach(count/s) : Outport
  wires:
  Floor3/1 -> back to rads/1
  to datatype limit/1 -> Floor3/1
  back to rads/1 -> to counts/1
  wm (rad/s)/1 -> to datatype limit/1
  Constant3/1 -> MATLAB Function2/2(t)
  to counts/1 -> tach(count/s)/1

== system Aero2_Workspace/Virtual Aero/Quantization, Noise, Datatypes, etc./Tachometer: Motor 1 ==
  wm (rad/s) : Inport
  Floor3 : Rounding
  back to rads : Gain  Gain=1/2^24
  to counts : Gain  Gain=4*512/(2*pi)
  to datatype limit : Gain  Gain=2^24
  tach(count/s) : Outport
  wires:
  wm (rad/s)/1 -> to datatype limit/1
  back to rads/1 -> to counts/1
  to datatype limit/1 -> Floor3/1
  Floor3/1 -> back to rads/1
  to counts/1 -> tach(count/s)/1

== system Aero2_Workspace/Virtual Aero/Quantization, Noise, Datatypes, etc./Tachometer: Pitch ==
  theta_dot (rad/s) : Inport
  Floor3 : Rounding
  Pitch: Rad to counts1 : Gain  Gain=4*720/(2*pi)
  back to rads : Gain  Gain=1/2^24
  to datatype limit : Gain  Gain=2^24
  tach (count/s) : Outport
  wires:
  theta_dot (rad/s)/1 -> to datatype limit/1
  back to rads/1 -> Pitch: Rad to counts1/1
  to datatype limit/1 -> Floor3/1
  Floor3/1 -> back to rads/1
  Pitch: Rad to counts1/1 -> tach (count/s)/1

== system Aero2_Workspace/Virtual Aero/Quantization, Noise, Datatypes, etc./Tachometer: Yaw ==
  psi_dot (rad/s) : Inport
  Floor3 : Rounding
  Yaw: Rad to counts1 : Gain  Gain=4*1024/(2*pi)
  back to rads : Gain  Gain=1/2^24
  to datatype limit : Gain  Gain=2^24
  tach (count/s) : Outport
  wires:
  Floor3/1 -> back to rads/1
  back to rads/1 -> Yaw: Rad to counts1/1
  to datatype limit/1 -> Floor3/1
  psi_dot (rad/s)/1 -> to datatype limit/1
  Yaw: Rad to counts1/1 -> tach (count/s)/1

== system Aero2_Workspace/Virtual Aero/Thruster Model 0/Variable Drag ==
  note: (4.5e-5/400*u+3e-5)*u
      | $\mu_d(\omega_m)=\mu_{d,slope}\omega_m+\mu_{d0}$
  wm (rad/s) : Inport
  Abs : Abs  SaturateOnIntegerOverflow=off
  Add : Sum
  mu_d * wm : Product
  mu_d slope : Gain  Gain=4.5e-5/400
  mu_do : Constant  Value=3e-5
  drag (N-m) : Outport
  wires:
  mu_do/1 -> Add/2
  mu_d * wm/1 -> drag (N-m)/1
  mu_d slope/1 -> Add/1
  Add/1 -> mu_d * wm/2
  wm (rad/s)/1 -> Abs/1, mu_d * wm/1
  Abs/1 -> mu_d slope/1

== system Aero2_Workspace/Virtual Aero/Thruster Model 1/Variable Drag ==
  note: (4.5e-5/400*u+3e-5)*u
      | $\mu_d(\omega_m)=\mu_{d,slope}\omega_m+\mu_{d0}$
  wm (rad/s) : Inport
  Abs : Abs  SaturateOnIntegerOverflow=off
  Add : Sum
  mu_d * wm : Product
  mu_d slope : Gain  Gain=4.5e-5/400
  mu_do : Constant  Value=3e-5
  drag (N-m) : Outport
  wires:
  wm (rad/s)/1 -> mu_d * wm/1, Abs/1
  Add/1 -> mu_d * wm/2
  mu_d slope/1 -> Add/1
  mu_d * wm/1 -> drag (N-m)/1
  mu_do/1 -> Add/2
  Abs/1 -> mu_d slope/1

== matlab function Aero2_Workspace/Virtual Aero/Quantization, Noise, Datatypes, etc./Tachometer: Motor 0/MATLAB Function2 ==
  data: u input; y output; t input
function y = tach_model(u, t)

y = u;

if (u >= 0)&&(u < t)
    y = t;
elseif (u < 0)&&(u > -t)
    y = -t;
end

== matlab function Aero2_Workspace/To//From Simulation1/MATLAB Function ==
  settings: updateMethod=DISCRETE  sampleTime=qc_get_step_size
  data: Packet output size=65537; ServerState input; SendStateUpdate input; DeviceNumber input; Pitch input; Yaw input; Enable output; Motor0Speed input; Motor1Speed input; BaseColor_v3 input
function [Packet,Enable] = Aero2MakePacket(ServerState, SendStateUpdate, DeviceNumber, Pitch, Yaw, Motor0Speed, Motor1Speed, BaseColor_v3) 

% Be sure to set the maximum signal size of the variable size Packet port 
% in Simulink->Edit Data of the editor window.  Size should be 65537 or
% larger to ensure that the stream server generates a 4 byte packet size.

%% Setup
persistent LastServerState;

if isempty(LastServerState)
    LastServerState = uint8(0);
end

Enable = 0;
Packet = uint8([]);

%% On connection
if ((ServerState == 2) && (LastServerState ~= 2))
    Packet = Aero2MakeCommandStateContainer(DeviceNumber, Yaw, Pitch, Motor0Speed, Motor1Speed, BaseColor_v3); 
    Packet = [Packet; Aero2MakeModeRequestContainer(DeviceNumber)];
end

%% Send new State Container
% Previous state processed, send a new one
if (SendStateUpdate)
    Packet = Aero2MakeCommandStateContainer(DeviceNumber, Yaw, Pitch, Motor0Speed, Motor1Speed, BaseColor_v3); 
   
end

%% Transmit
% If we have data to send, enable the transmit
PacketLength = length(Packet);

if (PacketLength > 0)
    % Add magic byte.  This is just for error handling and isn't typically
    % required in simulink, but useful in lower-level languages like Python
    Packet = [uint8(123); Packet];
    
    Enable = 1; 
end


LastServerState = ServerState;

== matlab function Aero2_Workspace/To//From Simulation1/MATLAB Function1 ==
  data: Receive input size=65537; RequestServerUpdate output; New input; YawLocked output double; PitchLocked output; HeliMode output; PropMode output double; Reset output; WeightOffset0 output double; WeightOffset1 output double
function [RequestServerUpdate, YawLocked, PitchLocked, HeliMode, PropMode, Reset, WeightOffset0, WeightOffset1]  = Aero2DecodePacket(Receive, New)

%% Setup

persistent iYawLocked;
persistent iPitchLocked;
persistent iHeliMode;
persistent iPropMode;
persistent iWeightOffset0;
persistent iWeightOffset1;

if isempty(iYawLocked)
    iYawLocked = uint8(0);
    iPitchLocked = uint8(0);
    iHeliMode = uint8(0);
    iPropMode = uint8(0);
    iWeightOffset0 = single(0);
    iWeightOffset1 = single(0);
end

% Need to assign outputs here even though they are reassigned at the end
% since matlab can't determine the signal widths
YawLocked = 0;
PitchLocked = 0;
HeliMode = 0;
PropMode = 0;
Reset = 0;
WeightOffset0 = 0;
WeightOffset1 = 0;

RequestServerUpdate = 0;
PacketSize = length(Receive);

% Packet > 0, new data, and magic number in first index
if ((PacketSize > 0) && (New == 1) && (Receive(1) == uint8(123)))
    
    %skip magic number
    Index = int32(2);
    
    while(Index <= PacketSize)
       
        %% Get container details
        ContainerSize = typecast(uint8(flip(Receive(Index:Index+3))), 'int32');
        ClassID = typecast(uint8(flip(Receive(Index+4:Index+7))), 'int32');
        DeviceNum = typecast(uint8(flip(Receive(Index+8:Index+11))), 'int32');
        DeviceFunction = uint8(Receive(Index+12));
        PayloadStart = Index+13;
        PayloadEnd = Index+ContainerSize-1;
        
        %% Pass container to appropriate decoding function
        if (ClassID == 91) %is this an Aero 2 container?
            
            if (DeviceFunction == 11) %UE4 State Response
                [iWeightOffset0, iWeightOffset1] = Aero2DecodeCommandAckContainer(Receive, PayloadStart);
                RequestServerUpdate = 1;
            elseif (DeviceFunction == 13) %Mode change
                [iYawLocked, iPitchLocked, iHeliMode, iPropMode] = Aero2DecodeModeContainer(Receive, PayloadStart);  
            end
        
        elseif (ClassID == 1001) %Simulink notification
            if (DeviceFunction == 200) %Reset button
                Reset = 1;
            end
        end
        
        
        
        %% Process next container if any data is left.
        Index = Index+ContainerSize;
    end


end

YawLocked = cast(iYawLocked, 'double');
PitchLocked = cast(iPitchLocked, 'double');
HeliMode = cast(iHeliMode, 'double');
PropMode = cast(iPropMode, 'double');
WeightOffset0 = cast(iWeightOffset0, 'double');
WeightOffset1 = cast(iWeightOffset1, 'double');
